simulink model "TeixeiraModel"  (R2015b)
settings: Solver=ode45  StartTime=0.0  StopTime=10.0  RelTol=1e-3
values from neighbouring files (symbols this model uses):
  C = [ ... (first row only)    [intrusionDetectionMS.m]
  F = A+H*C*L-k1*C    [intrusionDetectionMS.m]
  f1Val = 10    [intrusionDetectionMS.m]
  f2Val = 10    [intrusionDetectionMS.m]
  f3Val = 10    [intrusionDetectionMS.m]
  f4Val = 10    [intrusionDetectionMS.m]
  f5Val = 10    [intrusionDetectionMS.m]
  f6Val = 10    [intrusionDetectionMS.m]
  f7Val = 10    [intrusionDetectionMS.m]
  flt1 = 0    [intrusionDetectionMS.m]
  flt2 = 0    [intrusionDetectionMS.m]
  flt3 = 0    [intrusionDetectionMS.m]
  flt4 = 1    [intrusionDetectionMS.m]
  flt5 = 0    [intrusionDetectionMS.m]
  flt6 = 0    [intrusionDetectionMS.m]
  flt7 = 0    [intrusionDetectionMS.m]
  H = bf*CEin*CE'    [intrusionDetectionMS.m]
  k = k1 + F*H    [intrusionDetectionMS.m]
  L = [ ... (first row only)    [intrusionDetectionMS.m]
  tf1 = 2    [intrusionDetectionMS.m]
  tf2 = 2    [intrusionDetectionMS.m]
  tf3 = 2    [intrusionDetectionMS.m]
  tf4 = 2    [intrusionDetectionMS.m]
  tf5 = 2    [intrusionDetectionMS.m]
  tf6 = 5    [intrusionDetectionMS.m]
  tf7 = 7    [intrusionDetectionMS.m]
  x0 = [0 1 1 0 0 0 0]    [intrusionDetectionMS.m]
settings Model: Creator=sqn4594  LastModifiedBy=samnazari
settings DataIOCC: SaveFormat=Array
settings DebuggingCC: SolverPrmCheckMsg=warning  FcnCallInpInsideContextMsg=EnableAllAsWarning
settings HardwareCC: ProdBitPerPointer=32  ProdLargestAtomicFloat=None  ProdIntDivRoundTo=Undefined  ProdEndianess=Unspecified  ProdWordSize=32  ProdHWDeviceType=32-bit Generic
settings GRTTargetCC: GeneratePreprocessorConditionals=Disable all
settings ConfigComp: CovModelRefEnable=Off

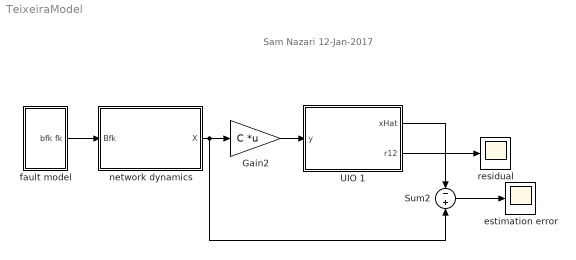
== system TeixeiraModel ==
  note: Sam Nazari
      | 12-Jan-2017
  Gain2 : Gain  Gain=C  Multiplication=Matrix(K*u)
  Sum2 : Sum  Inputs=-+
  UIO 1 : Subsystem
  estimation error : Scope
  fault model : Subsystem
  network dynamics : Subsystem
  residual : Scope
  wires:
  fault model/1(bfk fk) -> network dynamics/1(Bfk)
  network dynamics/1(X) -> Sum2/2, Gain2/1
  UIO 1/1("xHat ") -> Sum2/1
  Sum2/1 -> estimation error/1
  Gain2/1 -> UIO 1/1(y)
  UIO 1/2(r12) -> residual/1

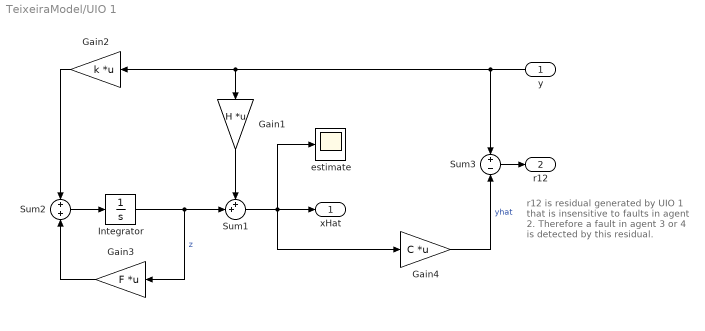
== system TeixeiraModel/UIO 1 ==
  note: r12 is residual generated by
      | UIO 1 that is insensitive to
      | faults in agent 2. Therefore a
      | fault in agent 3 or 4 is detected by
      | this residual.
  y : Inport
  Gain1 : Gain  Gain=H  Multiplication=Matrix(K*u)
  Gain2 : Gain  Gain=k  Multiplication=Matrix(K*u)
  Gain3 : Gain  Gain=F  Multiplication=Matrix(K*u)
  Gain4 : Gain  Gain=C  Multiplication=Matrix(K*u)
  Integrator : Integrator  InitialCondition=x0
  Sum1 : Sum  Inputs=++|
  Sum2 : Sum
  Sum3 : Sum  Inputs=+-
  estimate : Scope
  "xHat " : Outport
  r12 : Outport  Port=2
  wires:
  y/1 -> Gain1/1, Gain2/1, Sum3/1
  Sum2/1 -> Integrator/1
  Integrator/1 -> Sum1/2, Gain3/1  "z"
  Gain2/1 -> Sum2/1
  Gain3/1 -> Sum2/2
  Gain1/1 -> Sum1/1
  Sum1/1 -> Gain4/1, estimate/1, "xHat "/1
  Gain4/1 -> Sum3/2  "yhat"
  Sum3/1 -> r12/1

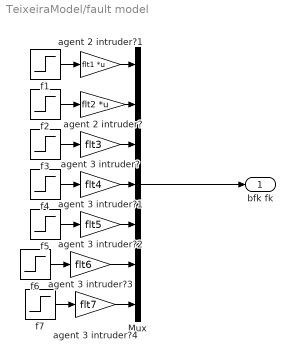
== system TeixeiraModel/fault model ==
  Mux : Mux  Inputs=7
  agent 2 intruder? : Gain  Gain=flt2  Multiplication=Matrix(K*u)
  agent 2 intruder?1 : Gain  Gain=flt1  Multiplication=Matrix(K*u)
  agent 3 intruder? : Gain  Gain=flt3
  agent 3 intruder?1 : Gain  Gain=flt4
  agent 3 intruder?2 : Gain  Gain=flt5
  agent 3 intruder?3 : Gain  Gain=flt6
  agent 3 intruder?4 : Gain  Gain=flt7
  f1 : Step  After=f1Val  SampleTime=tf1
  f2 : Step  After=f2Val  SampleTime=tf2
  f3 : Step  After=f3Val  SampleTime=tf3
  f4 : Step  After=f4Val  SampleTime=tf4
  f5 : Step  After=f5Val  SampleTime=tf5
  f6 : Step  After=f6Val  SampleTime=tf6
  f7 : Step  After=f7Val  SampleTime=tf7
  bfk fk : Outport
  wires:
  Mux/1 -> bfk fk/1
  f1/1 -> agent 2 intruder?1/1
  f2/1 -> agent 2 intruder?/1
  f3/1 -> agent 3 intruder?/1
  agent 2 intruder?/1 -> Mux/2
  agent 3 intruder?/1 -> Mux/3
  agent 2 intruder?1/1 -> Mux/1
  f4/1 -> agent 3 intruder?1/1
  agent 3 intruder?1/1 -> Mux/4
  agent 3 intruder?2/1 -> Mux/5
  f5/1 -> agent 3 intruder?2/1
  f6/1 -> agent 3 intruder?3/1
  agent 3 intruder?3/1 -> Mux/6
  f7/1 -> agent 3 intruder?4/1
  agent 3 intruder?4/1 -> Mux/7

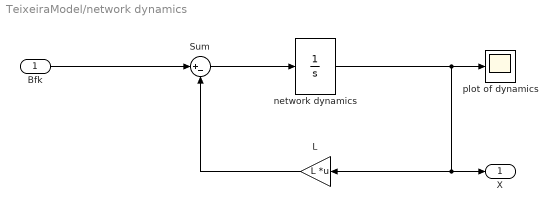
== system TeixeiraModel/network dynamics ==
  Bfk : Inport
  L : Gain  Gain=L  Multiplication=Matrix(K*u)
  Sum : Sum  Inputs=|+-
  network dynamics : Integrator  InitialCondition=x0
  plot of dynamics : Scope
  X : Outport
  wires:
  Bfk/1 -> Sum/1
  Sum/1 -> network dynamics/1
  network dynamics/1 -> plot of dynamics/1, X/1, L/1
  L/1 -> Sum/2
